simulink model "TestCoupleNew"  (R2024b)
settings: Solver=ode45  StartTime=0.0  StopTime=TimeTqStop  MaxStep=0.1  RelTol=1e-3  EnableMultiTasking=on
undefined symbols (not defined in the file): AAopti, AATq, Copti, PcolTq, RegimeTq, table_rdt_AA, TempsTq, TorqueTest, TorqueTimeTest, Vcyl, vect_delta_AA
settings Model: Creator=a030141  LastModifiedBy=ramse
settings SolverCC: AlgebraicLoopSolver=TrustRegion
settings DataIOCC: LimitDataPoints=on  SaveFormat=Array  SignalLoggingSaveFormat=ModelDataLogs  ReturnWorkspaceOutputs=off  SignalLoggingName=sigsOut
settings OptimizationCC: InitFltsAndDblsToZero=on  LifeSpan=inf
settings DebuggingCC: SaveWithParameterizedLinksMsg=none  UnderspecifiedInitializationDetection=Classic  MergeDetectMultiDrivingBlocksExec=none  SignalResolutionControl=TryResolveAllWithWarning  MultiTaskDSMMsg=warning  MultiTaskCondExecSysMsg=none  FcnCallInpInsideContextMsg=warning  UnconnectedInputMsg=warning  UnconnectedOutputMsg=warning  UnconnectedLineMsg=warning  SFUnexpectedBacktrackingDiag=warning  SFNoUnconditionalDefaultTransitionDiag=warning  SFExecutionAtInitializationDiag=none  ArithmeticOperatorsInVariantConditions=warning
settings HardwareCC: ProdBitPerPointer=32  ProdBitPerSizeT=32  ProdBitPerPtrDiffT=32  ProdLargestAtomicFloat=None  ProdIntDivRoundTo=Undefined  ProdEndianess=Unspecified  ProdWordSize=32  ProdHWDeviceType=32-bit Generic  TargetBitPerPointer=64  TargetBitPerSizeT=64  TargetBitPerPtrDiffT=64  TargetLongLongMode=on  TargetIntDivRoundTo=Zero  TargetEndianess=LittleEndian  TargetWordSize=64  TargetHWDeviceType=MATLAB Host  ProdEqTarget=off
settings ModelReferenceCC: PropagateSignalLabelsOutOfModel=off
settings RTWCC: GPUComputeCapability=3.5
settings CodeAppCC: StateflowObjectComments=on
settings GRTTargetCC: TargetFcnLib=ansi_tfl_tmw.mat  TargetLangStandard=C89/C90 (ANSI)  CombineOutputUpdateFcns=off  GRTInterface=on
settings ConfigComp: CovMetricSettings=dw  CovSaveCumulativeToWorkspaceVar=on  CovSaveSingleToWorkspaceVar=on

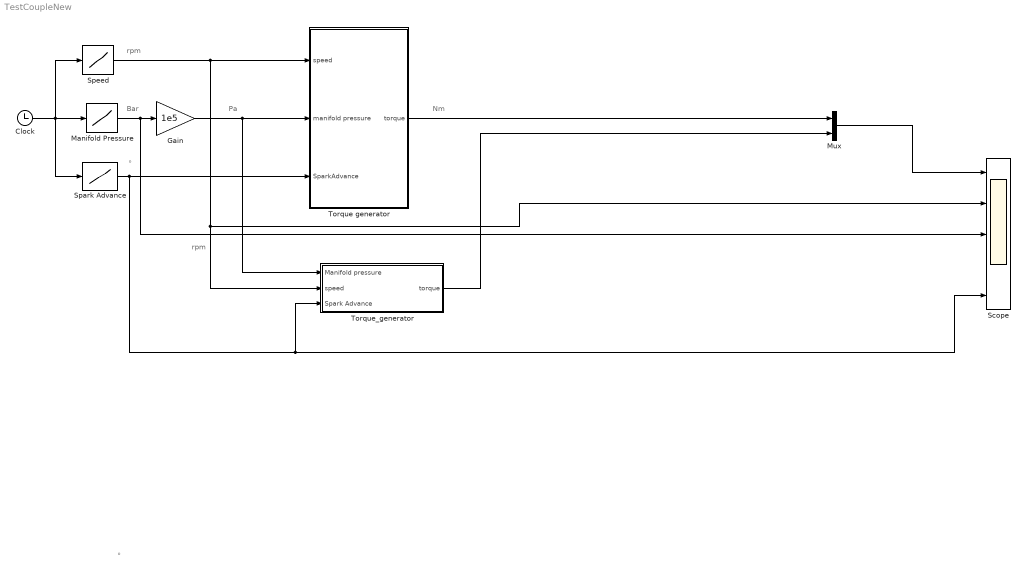
== system TestCoupleNew ==
  note: Nm
  note: Bar
  note: °
  note: rpm
  note: Pa
  note: rpm
  note: °
  Clock : Clock
  Gain : Gain  Gain=1e5  SaturateOnIntegerOverflow=on  OutDataTypeStr=Inherit: Same as input  ParamDataTypeStr=Inherit: Same as input
  Manifold Pressure : Lookup  InputValues=TempsTq  Table=PcolTq
  Mux : Mux  Inputs=2
  Scope : Scope  NumInputPorts=5
  Spark Advance : Lookup  InputValues=TempsTq  Table=AATq
  Speed : Lookup  InputValues=TempsTq  Table=RegimeTq
  Torque generator : Subsystem
  Torque_generator : Subsystem
  wires:
  Clock/1 -> Spark Advance/1, Manifold Pressure/1, Speed/1
  Spark Advance/1 -> Torque_generator/3(Spark Advance), Scope/5, Torque generator/3(SparkAdvance)
  Mux/1 -> Scope/1
  Gain/1 -> Torque_generator/1(Manifold pressure), Torque generator/2(manifold pressure)
  Manifold Pressure/1 -> Scope/3, Gain/1
  Speed/1 -> Torque_generator/2(speed), Scope/2, Torque generator/1(speed)
  Torque generator/1(torque) -> Mux/1
  Torque_generator/1(torque) -> Mux/2

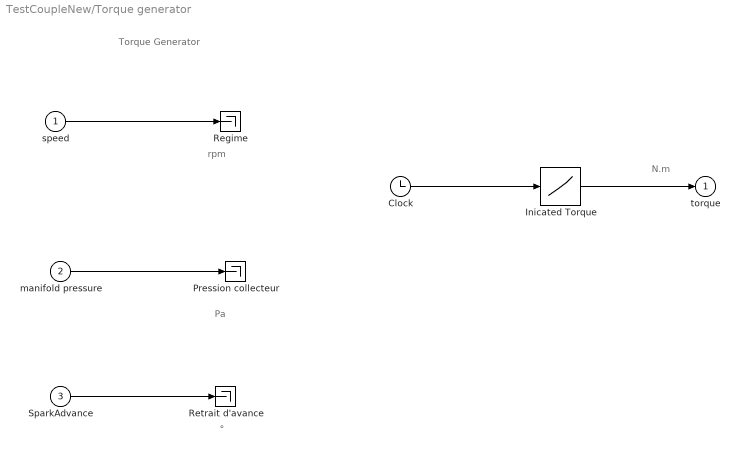
== system TestCoupleNew/Torque generator ==
  note: Torque Generator
  note: N.m
  note: rpm
  note: Pa
  note: °
  speed : Inport
  manifold pressure : Inport  Port=2
  SparkAdvance : Inport  Port=3
  Clock : Clock
  Inicated Torque : Lookup  InputValues=TorqueTimeTest  Table=TorqueTest
  Pression collecteur : Terminator
  Regime : Terminator
  Retrait d'avance : Terminator
  torque : Outport
  wires:
  Inicated Torque/1 -> torque/1
  speed/1 -> Regime/1
  SparkAdvance/1 -> Retrait d'avance/1
  manifold pressure/1 -> Pression collecteur/1
  Clock/1 -> Inicated Torque/1

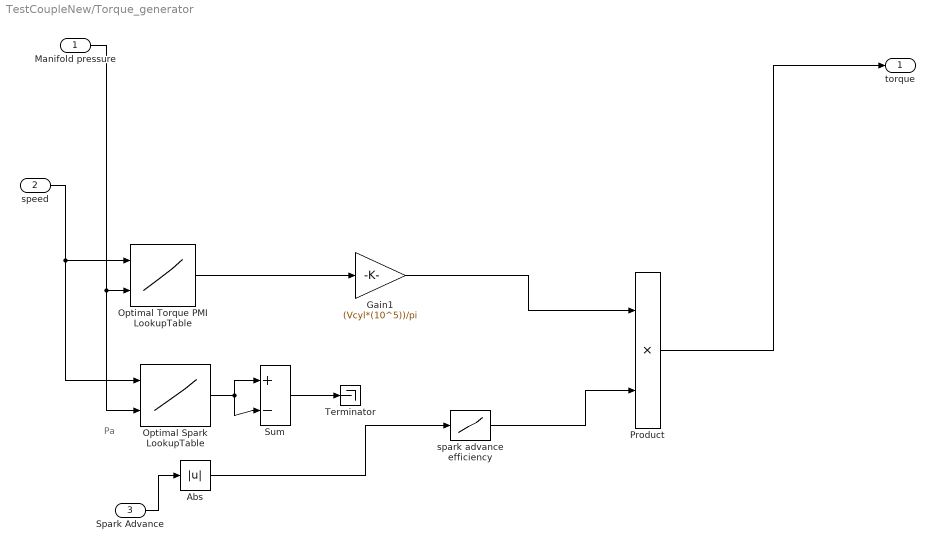
== system TestCoupleNew/Torque_generator ==
  note: Pa
  Manifold pressure : Inport
  speed : Inport  Port=2
  Spark Advance : Inport  Port=3
  Abs : Abs  SaturateOnIntegerOverflow=off
  Gain1 : Gain  Gain=(Vcyl*(10^5))/pi
  Optimal Spark LookupTable : Lookup2D  RowIndex=Ne_remp  ColumnIndex=Pcol_remp  Table=AAopti
  Optimal Torque PMI LookupTable : Lookup2D  RowIndex=Ne_remp  ColumnIndex=Pcol_remp  Table=Copti
  Product : Product
  Sum : Sum  Inputs=|+-
  Terminator : Terminator
  spark advance efficiency : Lookup  InputValues=vect_delta_AA  Table=table_rdt_AA
  torque : Outport
  wires:
  spark advance efficiency/1 -> Product/2
  speed/1 -> Optimal Spark LookupTable/1, Optimal Torque PMI LookupTable/1
  Gain1/1 -> Product/1
  Abs/1 -> spark advance efficiency/1
  Optimal Spark LookupTable/1 -> Sum/2, Sum/1
  Optimal Torque PMI LookupTable/1 -> Gain1/1
  Manifold pressure/1 -> Optimal Spark LookupTable/2, Optimal Torque PMI LookupTable/2
  Sum/1 -> Terminator/1
  Product/1 -> torque/1
  Spark Advance/1 -> Abs/1
